simulink model "sysgenImageDoubleBuffer"  (Simulink 7.7)
settings: Solver=VariableStepDiscrete  StartTime=0.0  StopTime=((c_rx_rows_2*c_rx_cols_2)*2+(320*10))+5000  RelTol=1e-3
PreLoadFcn:
  | sysgenImageDoubleBuffer_PreLoadFcn
StartFcn:
  | tic;
undefined symbols (not defined in the file or in its folder): c_rx_cols_1, c_rx_cols_2, c_rx_rows_1, c_rx_rows_2, dpost_1, dpost_2
libraries: xbsIndex_r4 x160, dspbuff3 x6, dspsigattribs x6, dspmtrx3 x6, vipsrcs x2, simulink x2, xbsCopyrightNotice_r4 x1
(part 3 of 3)

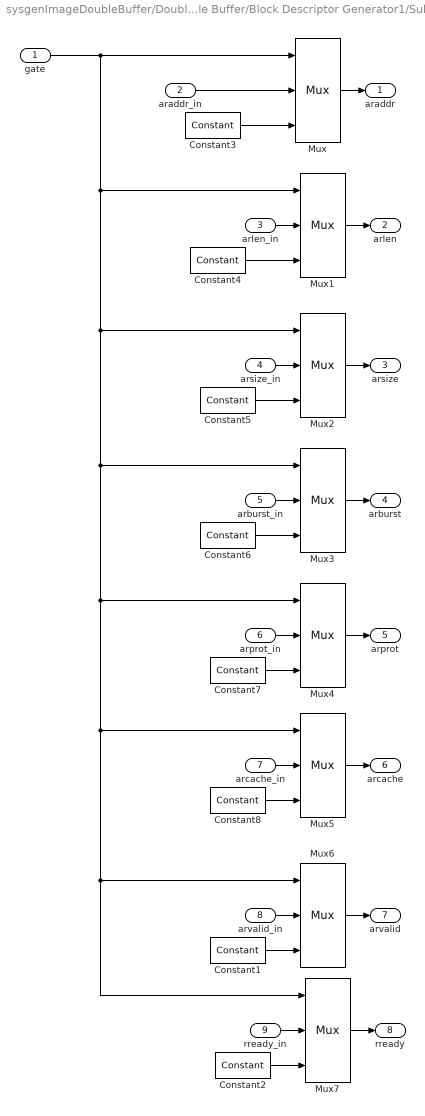
== system sysgenImageDoubleBuffer/Double Buffer/Double Buffer/Block Descriptor Generator1/Subsystem ==
  gate : Inport
  araddr_in : Inport  Port=2
  arlen_in : Inport  Port=3
  arsize_in : Inport  Port=4
  arburst_in : Inport  Port=5
  arprot_in : Inport  Port=6
  arcache_in : Inport  Port=7
  arvalid_in : Inport  Port=8
  rready_in : Inport  Port=9
  Constant1 : xbsIndex_r4/Constant  const=0  gui_display_data_type=Fixed-point  arith_type=Boolean  n_bits=4  bin_pt=0  preci_type=Single  exp_width=8  frac_width=24  explicit_period=off  period=1  equ=P=C  opselect=C  inp2=PCIN>>17  opr=+  inp1=P  carry=CIN  dbl_ovrd=off  block_type=constant
      settings: block_version=12.3
  Constant2 : xbsIndex_r4/Constant  const=0  gui_display_data_type=Fixed-point  arith_type=Boolean  n_bits=4  bin_pt=0  preci_type=Single  exp_width=8  frac_width=24  explicit_period=off  period=1  equ=P=C  opselect=C  inp2=PCIN>>17  opr=+  inp1=P  carry=CIN  dbl_ovrd=off  block_type=constant
      settings: block_version=12.3
  Constant3 : xbsIndex_r4/Constant  const=0  gui_display_data_type=Fixed-point  arith_type=Unsigned  n_bits=32  bin_pt=0  preci_type=Single  exp_width=8  frac_width=24  explicit_period=off  period=1  equ=P=C  opselect=C  inp2=PCIN>>17  opr=+  inp1=P  carry=CIN  dbl_ovrd=off  block_type=constant
      settings: block_version=12.3
  Constant4 : xbsIndex_r4/Constant  const=0  gui_display_data_type=Fixed-point  arith_type=Unsigned  n_bits=8  bin_pt=0  preci_type=Single  exp_width=8  frac_width=24  explicit_period=off  period=1  equ=P=C  opselect=C  inp2=PCIN>>17  opr=+  inp1=P  carry=CIN  dbl_ovrd=off  block_type=constant
      settings: block_version=12.3
  Constant5 : xbsIndex_r4/Constant  const=0  gui_display_data_type=Fixed-point  arith_type=Unsigned  n_bits=3  bin_pt=0  preci_type=Single  exp_width=8  frac_width=24  explicit_period=off  period=1  equ=P=C  opselect=C  inp2=PCIN>>17  opr=+  inp1=P  carry=CIN  dbl_ovrd=off  block_type=constant
      settings: block_version=12.3
  Constant6 : xbsIndex_r4/Constant  const=0  gui_display_data_type=Fixed-point  arith_type=Unsigned  n_bits=2  bin_pt=0  preci_type=Single  exp_width=8  frac_width=24  explicit_period=off  period=1  equ=P=C  opselect=C  inp2=PCIN>>17  opr=+  inp1=P  carry=CIN  dbl_ovrd=off  block_type=constant
      settings: block_version=12.3
  Constant7 : xbsIndex_r4/Constant  const=0  gui_display_data_type=Fixed-point  arith_type=Unsigned  n_bits=3  bin_pt=0  preci_type=Single  exp_width=8  frac_width=24  explicit_period=off  period=1  equ=P=C  opselect=C  inp2=PCIN>>17  opr=+  inp1=P  carry=CIN  dbl_ovrd=off  block_type=constant
      settings: block_version=12.3
  Constant8 : xbsIndex_r4/Constant  const=0  gui_display_data_type=Fixed-point  arith_type=Unsigned  n_bits=4  bin_pt=0  preci_type=Single  exp_width=8  frac_width=24  explicit_period=off  period=1  equ=P=C  opselect=C  inp2=PCIN>>17  opr=+  inp1=P  carry=CIN  dbl_ovrd=off  block_type=constant
      settings: block_version=12.3
  Mux{,1..7} (8 alike) : xbsIndex_r4/Mux  inputs=2  en=off  latency=0  precision=Full  arith_type=Unsigned  n_bits=16  bin_pt=14  quantization=Truncate  overflow=Wrap  dbl_ovrd=off  block_type=mux
      settings: block_version=12.3
  araddr : Outport
  arlen : Outport  Port=2
  arsize : Outport  Port=3
  arburst : Outport  Port=4
  arprot : Outport  Port=5
  arcache : Outport  Port=6
  arvalid : Outport  Port=7
  rready : Outport  Port=8
  wires:
  Constant3/1 -> Mux/3
  Constant4/1 -> Mux1/3
  Constant5/1 -> Mux2/3
  Constant6/1 -> Mux3/3
  Constant7/1 -> Mux4/3
  Constant8/1 -> Mux5/3
  gate/1 -> Mux/1, Mux1/1, Mux2/1, Mux3/1, Mux4/1, Mux5/1, Mux6/1, Mux7/1
  araddr_in/1 -> Mux/2
  Mux/1 -> araddr/1
  arlen_in/1 -> Mux1/2
  Mux1/1 -> arlen/1
  arsize_in/1 -> Mux2/2
  Mux2/1 -> arsize/1
  arburst_in/1 -> Mux3/2
  Mux3/1 -> arburst/1
  arprot_in/1 -> Mux4/2
  Mux4/1 -> arprot/1
  arcache_in/1 -> Mux5/2
  Mux5/1 -> arcache/1
  Constant1/1 -> Mux6/3
  arvalid_in/1 -> Mux6/2
  Mux6/1 -> arvalid/1
  Constant2/1 -> Mux7/3
  rready_in/1 -> Mux7/2
  Mux7/1 -> rready/1

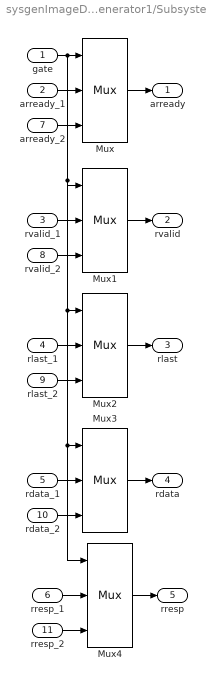
== system sysgenImageDoubleBuffer/Double Buffer/Double Buffer/Block Descriptor Generator1/Subsystem1 ==
  gate : Inport
  arready_1 : Inport  Port=2
  rvalid_1 : Inport  Port=3
  rlast_1 : Inport  Port=4
  rdata_1 : Inport  Port=5
  rresp_1 : Inport  Port=6
  arready_2 : Inport  Port=7
  rvalid_2 : Inport  Port=8
  rlast_2 : Inport  Port=9
  rdata_2 : Inport  Port=10
  rresp_2 : Inport  Port=11
  Mux{,1..4} (5 alike) : xbsIndex_r4/Mux  inputs=2  en=off  latency=0  precision=Full  arith_type=Unsigned  n_bits=16  bin_pt=14  quantization=Truncate  overflow=Wrap  dbl_ovrd=off  block_type=mux
      settings: block_version=12.3
  arready : Outport
  rvalid : Outport  Port=2
  rlast : Outport  Port=3
  rdata : Outport  Port=4
  rresp : Outport  Port=5
  wires:
  gate/1 -> Mux/1, Mux1/1, Mux2/1, Mux3/1, Mux4/1
  arready_1/1 -> Mux/2
  Mux/1 -> arready/1
  arready_2/1 -> Mux/3
  rvalid_1/1 -> Mux1/2
  Mux1/1 -> rvalid/1
  rvalid_2/1 -> Mux1/3
  rlast_1/1 -> Mux2/2
  Mux2/1 -> rlast/1
  rlast_2/1 -> Mux2/3
  rdata_1/1 -> Mux3/2
  Mux3/1 -> rdata/1
  rdata_2/1 -> Mux3/3
  rresp_1/1 -> Mux4/2
  Mux4/1 -> rresp/1
  rresp_2/1 -> Mux4/3

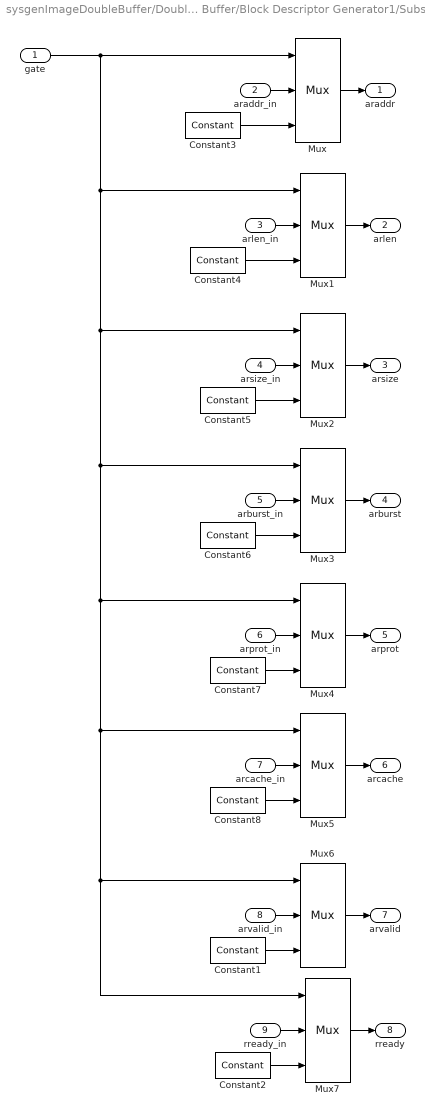
== system sysgenImageDoubleBuffer/Double Buffer/Double Buffer/Block Descriptor Generator1/Subsystem4 ==
  gate : Inport
  araddr_in : Inport  Port=2
  arlen_in : Inport  Port=3
  arsize_in : Inport  Port=4
  arburst_in : Inport  Port=5
  arprot_in : Inport  Port=6
  arcache_in : Inport  Port=7
  arvalid_in : Inport  Port=8
  rready_in : Inport  Port=9
  Constant1 : xbsIndex_r4/Constant  const=0  gui_display_data_type=Fixed-point  arith_type=Boolean  n_bits=4  bin_pt=0  preci_type=Single  exp_width=8  frac_width=24  explicit_period=off  period=1  equ=P=C  opselect=C  inp2=PCIN>>17  opr=+  inp1=P  carry=CIN  dbl_ovrd=off  block_type=constant
      settings: block_version=12.3
  Constant2 : xbsIndex_r4/Constant  const=0  gui_display_data_type=Fixed-point  arith_type=Boolean  n_bits=4  bin_pt=0  preci_type=Single  exp_width=8  frac_width=24  explicit_period=off  period=1  equ=P=C  opselect=C  inp2=PCIN>>17  opr=+  inp1=P  carry=CIN  dbl_ovrd=off  block_type=constant
      settings: block_version=12.3
  Constant3 : xbsIndex_r4/Constant  const=0  gui_display_data_type=Fixed-point  arith_type=Unsigned  n_bits=32  bin_pt=0  preci_type=Single  exp_width=8  frac_width=24  explicit_period=off  period=1  equ=P=C  opselect=C  inp2=PCIN>>17  opr=+  inp1=P  carry=CIN  dbl_ovrd=off  block_type=constant
      settings: block_version=12.3
  Constant4 : xbsIndex_r4/Constant  const=0  gui_display_data_type=Fixed-point  arith_type=Unsigned  n_bits=8  bin_pt=0  preci_type=Single  exp_width=8  frac_width=24  explicit_period=off  period=1  equ=P=C  opselect=C  inp2=PCIN>>17  opr=+  inp1=P  carry=CIN  dbl_ovrd=off  block_type=constant
      settings: block_version=12.3
  Constant5 : xbsIndex_r4/Constant  const=0  gui_display_data_type=Fixed-point  arith_type=Unsigned  n_bits=3  bin_pt=0  preci_type=Single  exp_width=8  frac_width=24  explicit_period=off  period=1  equ=P=C  opselect=C  inp2=PCIN>>17  opr=+  inp1=P  carry=CIN  dbl_ovrd=off  block_type=constant
      settings: block_version=12.3
  Constant6 : xbsIndex_r4/Constant  const=0  gui_display_data_type=Fixed-point  arith_type=Unsigned  n_bits=2  bin_pt=0  preci_type=Single  exp_width=8  frac_width=24  explicit_period=off  period=1  equ=P=C  opselect=C  inp2=PCIN>>17  opr=+  inp1=P  carry=CIN  dbl_ovrd=off  block_type=constant
      settings: block_version=12.3
  Constant7 : xbsIndex_r4/Constant  const=0  gui_display_data_type=Fixed-point  arith_type=Unsigned  n_bits=3  bin_pt=0  preci_type=Single  exp_width=8  frac_width=24  explicit_period=off  period=1  equ=P=C  opselect=C  inp2=PCIN>>17  opr=+  inp1=P  carry=CIN  dbl_ovrd=off  block_type=constant
      settings: block_version=12.3
  Constant8 : xbsIndex_r4/Constant  const=0  gui_display_data_type=Fixed-point  arith_type=Unsigned  n_bits=4  bin_pt=0  preci_type=Single  exp_width=8  frac_width=24  explicit_period=off  period=1  equ=P=C  opselect=C  inp2=PCIN>>17  opr=+  inp1=P  carry=CIN  dbl_ovrd=off  block_type=constant
      settings: block_version=12.3
  Mux{,1..7} (8 alike) : xbsIndex_r4/Mux  inputs=2  en=off  latency=0  precision=Full  arith_type=Unsigned  n_bits=16  bin_pt=14  quantization=Truncate  overflow=Wrap  dbl_ovrd=off  block_type=mux
      settings: block_version=12.3
  araddr : Outport
  arlen : Outport  Port=2
  arsize : Outport  Port=3
  arburst : Outport  Port=4
  arprot : Outport  Port=5
  arcache : Outport  Port=6
  arvalid : Outport  Port=7
  rready : Outport  Port=8
  wires:
  Mux7/1 -> rready/1
  rready_in/1 -> Mux7/2
  Constant2/1 -> Mux7/3
  Mux6/1 -> arvalid/1
  arvalid_in/1 -> Mux6/2
  Constant1/1 -> Mux6/3
  Mux5/1 -> arcache/1
  arcache_in/1 -> Mux5/2
  Mux4/1 -> arprot/1
  arprot_in/1 -> Mux4/2
  Mux3/1 -> arburst/1
  arburst_in/1 -> Mux3/2
  Mux2/1 -> arsize/1
  arsize_in/1 -> Mux2/2
  Mux1/1 -> arlen/1
  arlen_in/1 -> Mux1/2
  Mux/1 -> araddr/1
  araddr_in/1 -> Mux/2
  gate/1 -> Mux7/1, Mux6/1, Mux5/1, Mux4/1, Mux3/1, Mux2/1, Mux1/1, Mux/1
  Constant8/1 -> Mux5/3
  Constant7/1 -> Mux4/3
  Constant6/1 -> Mux3/3
  Constant5/1 -> Mux2/3
  Constant4/1 -> Mux1/3
  Constant3/1 -> Mux/3

== system sysgenImageDoubleBuffer/Image_Source_1/Image_source_1/Subsystem1/pixelize ==
  In1 : Inport
  Convert 2-D to 1-D : dspsigattribs/Convert 2-D to 1-D  SystemSampleTime=-1
  Frame Conversion : FrameConversion
  Transpose : dspmtrx3/Transpose  SystemSampleTime=-1  Hermitian=off  overflowFlag=off
  Unbuffer1 : Unbuffer
  Out1 : Outport
  wires:
  Convert 2-D to 1-D/1 -> Frame Conversion/1
  Frame Conversion/1 -> Unbuffer1/1
  Transpose/1 -> Convert 2-D to 1-D/1
  In1/1 -> Transpose/1
  Unbuffer1/1 -> Out1/1

== system sysgenImageDoubleBuffer/Image_Source_1/Image_source_1/Subsystem1/pixelize1 ==
  In1 : Inport
  Convert 2-D to 1-D : dspsigattribs/Convert 2-D to 1-D  SystemSampleTime=-1
  Frame Conversion : FrameConversion
  Transpose : dspmtrx3/Transpose  SystemSampleTime=-1  Hermitian=off  overflowFlag=off
  Unbuffer1 : Unbuffer
  Out1 : Outport
  wires:
  Unbuffer1/1 -> Out1/1
  In1/1 -> Transpose/1
  Transpose/1 -> Convert 2-D to 1-D/1
  Frame Conversion/1 -> Unbuffer1/1
  Convert 2-D to 1-D/1 -> Frame Conversion/1

== system sysgenImageDoubleBuffer/Image_Source_1/Image_source_1/Subsystem1/pixelize2 ==
  In1 : Inport
  Convert 2-D to 1-D : dspsigattribs/Convert 2-D to 1-D  SystemSampleTime=-1
  Frame Conversion : FrameConversion
  Transpose : dspmtrx3/Transpose  SystemSampleTime=-1  Hermitian=off  overflowFlag=off
  Unbuffer1 : Unbuffer
  Out1 : Outport
  wires:
  Convert 2-D to 1-D/1 -> Frame Conversion/1
  Frame Conversion/1 -> Unbuffer1/1
  Transpose/1 -> Convert 2-D to 1-D/1
  In1/1 -> Transpose/1
  Unbuffer1/1 -> Out1/1

== system sysgenImageDoubleBuffer/image_Source_2/image_source_2/Subsystem3/pixelize ==
  In1 : Inport
  Convert 2-D to 1-D : dspsigattribs/Convert 2-D to 1-D  SystemSampleTime=-1
  Frame Conversion : FrameConversion
  Transpose : dspmtrx3/Transpose  SystemSampleTime=-1  Hermitian=off  overflowFlag=off
  Unbuffer1 : Unbuffer
  Out1 : Outport
  wires:
  Convert 2-D to 1-D/1 -> Frame Conversion/1
  Frame Conversion/1 -> Unbuffer1/1
  Transpose/1 -> Convert 2-D to 1-D/1
  In1/1 -> Transpose/1
  Unbuffer1/1 -> Out1/1

== system sysgenImageDoubleBuffer/image_Source_2/image_source_2/Subsystem3/pixelize1 ==
  In1 : Inport
  Convert 2-D to 1-D : dspsigattribs/Convert 2-D to 1-D  SystemSampleTime=-1
  Frame Conversion : FrameConversion
  Transpose : dspmtrx3/Transpose  SystemSampleTime=-1  Hermitian=off  overflowFlag=off
  Unbuffer1 : Unbuffer
  Out1 : Outport
  wires:
  Unbuffer1/1 -> Out1/1
  In1/1 -> Transpose/1
  Transpose/1 -> Convert 2-D to 1-D/1
  Frame Conversion/1 -> Unbuffer1/1
  Convert 2-D to 1-D/1 -> Frame Conversion/1

== system sysgenImageDoubleBuffer/image_Source_2/image_source_2/Subsystem3/pixelize2 ==
  In1 : Inport
  Convert 2-D to 1-D : dspsigattribs/Convert 2-D to 1-D  SystemSampleTime=-1
  Frame Conversion : FrameConversion
  Transpose : dspmtrx3/Transpose  SystemSampleTime=-1  Hermitian=off  overflowFlag=off
  Unbuffer1 : Unbuffer
  Out1 : Outport
  wires:
  Convert 2-D to 1-D/1 -> Frame Conversion/1
  Frame Conversion/1 -> Unbuffer1/1
  Transpose/1 -> Convert 2-D to 1-D/1
  In1/1 -> Transpose/1
  Unbuffer1/1 -> Out1/1
